simulink model "FCS_MPC_6ph_Regelungsmodell"  (R2022a)
settings: Solver=ode23t  StartTime=0.0  StopTime=0.1  RelTol=1e-3  AbsTol=1e-3  EnableMultiTasking=on
values from neighbouring files (symbols this model uses):
  f_c = 100000    [MPC_params.m]
  L_d = 2e-3    (= 0.002)    [MPC_params.m]
  L_q = 6.4e-3    (= 0.0064)    [MPC_params.m]
  L_x = 3e-3    (= 0.003)    [MPC_params.m]
  L_y = L_x    (= 0.003)    [MPC_params.m]
  p = 5    [MPC_params.m]
  psi_pm = 0.19    [MPC_params.m]
  R_ph = 0.19    [MPC_params.m]
  T_100MHz = 1/f_100MHz    (= 1e-08)    [MPC_params.m]
  u_dc = 565    [MPC_params.m]
libraries: nesl_utility x39, fl_lib x32, ee_lib x12, simulink x4, hdlsllib x3, spsAlphaBetaZerotodq0Lib x1
(part 2 of 2)

== matlab function FCS_MPC_6ph_Regelungsmodell/Microcontroller Software/Subsystem5/MATLAB Function1 ==
  data: I input; next_switching_state output
function next_switching_state = fcn(I)

    % Possible switching states of the 6-Phase 2-level inverter
    possible_swichting_states = [0	1	0	1	0	1	0	1	0	1	0	1;
                                1	0	0	1	0	1	0	1	0	1	0	1;
                                0	1	1	0	0	1	0	1	0	1	0	1;
                                1	0	1	0	0	1	0	1	0	1	0	1;
                                0	1	0	1	1	0	0	1	0	1	0	1;
                                1	0	0	1	1	0	0	1	0	1	0	1;
                                0	1	1	0	1	0	0	1	0	1	0	1;
                                1	0	1	0	1	0	0	1	0	1	0	1;
                                0	1	0	1	0	1	1	0	0	1	0	1;
                                1	0	0	1	0	1	1	0	0	1	0	1;
                                0	1	1	0	0	1	1	0	0	1	0	1;
                                1	0	1	0	0	1	1	0	0	1	0	1;
                                0	1	0	1	1	0	1	0	0	1	0	1;
                                1	0	0	1	1	0	1	0	0	1	0	1;
                                0	1	1	0	1	0	1	0	0	1	0	1;
                                1	0	1	0	1	0	1	0	0	1	0	1;
                                0	1	0	1	0	1	0	1	1	0	0	1;
                                1	0	0	1	0	1	0	1	1	0	0	1;
                                0	1	1	0	0	1	0	1	1	0	0	1;
                                1	0	1	0	0	1	0	1	1	0	0	1;
                                0	1	0	1	1	0	0	1	1	0	0	1;
                                1	0	0	1	1	0	0	1	1	0	0	1;
                                0	1	1	0	1	0	0	1	1	0	0	1;
                                1	0	1	0	1	0	0	1	1	0	0	1;
                                0	1	0	1	0	1	1	0	1	0	0	1;
                                1	0	0	1	0	1	1	0	1	0	0	1;
                                0	1	1	0	0	1	1	0	1	0	0	1;
                                1	0	1	0	0	1	1	0	1	0	0	1;
                                0	1	0	1	1	0	1	0	1	0	0	1;
                                1	0	0	1	1	0	1	0	1	0	0	1;
                                0	1	1	0	1	0	1	0	1	0	0	1;
                                1	0	1	0	1	0	1	0	1	0	0	1;
                                0	1	0	1	0	1	0	1	0	1	1	0;
                                1	0	0	1	0	1	0	1	0	1	1	0;
                                0	1	1	0	0	1	0	1	0	1	1	0;
                                1	0	1	0	0	1	0	1	0	1	1	0;
                                0	1	0	1	1	0	0	1	0	1	1	0;
                                1	0	0	1	1	0	0	1	0	1	1	0;
                                0	1	1	0	1	0	0	1	0	1	1	0;
                                1	0	1	0	1	0	0	1	0	1	1	0;
                                0	1	0	1	0	1	1	0	0	1	1	0;
                                1	0	0	1	0	1	1	0	0	1	1	0;
                                0	1	1	0	0	1	1	0	0	1	1	0;
                                1	0	1	0	0	1	1	0	0	1	1	0;
                                0	1	0	1	1	0	1	0	0	1	1	0;
                                1	0	0	1	1	0	1	0	0	1	1	0;
                                0	1	1	0	1	0	1	0	0	1	1	0;
                                1	0	1	0	1	0	1	0	0	1	1	0;
                                0	1	0	1	0	1	0	1	1	0	1	0;
                                1	0	0	1	0	1	0	1	1	0	1	0;
                                0	1	1	0	0	1	0	1	1	0	1	0;
                                1	0	1	0	0	1	0	1	1	0	1	0;
                                0	1	0	1	1	0	0	1	1	0	1	0;
                                1	0	0	1	1	0	0	1	1	0	1	0;
                                0	1	1	0	1	0	0	1	1	0	1	0;
                                1	0	1	0	1	0	0	1	1	0	1	0;
                                0	1	0	1	0	1	1	0	1	0	1	0;
                                1	0	0	1	0	1	1	0	1	0	1	0;
                                0	1	1	0	0	1	1	0	1	0	1	0;
                                1	0	1	0	0	1	1	0	1	0	1	0;
                                0	1	0	1	1	0	1	0	1	0	1	0;
                                1	0	0	1	1	0	1	0	1	0	1	0;
                                0	1	1	0	1	0	1	0	1	0	1	0;
                                1	0	1	0	1	0	1	0	1	0	1	0];

    % Initial condition
    if I==0
        I=int32(1);
    end

    % Output switching state
    next_switching_state=boolean(possible_swichting_states(I,:))';

end

== matlab function FCS_MPC_6ph_Regelungsmodell/6ph_PMSM_30deg_VSD1 ==
  data: u1 input; y1 output; u2 input; u3 input; u4 input; u5 input; u6 input; y2 output; y3 output; y4 output; y5 output; y6 output; k6 input; c6 input
function [y1,y2,y3,y4,y5,y6] = VSD_asymm_30(u1,u2,u3,u4,u5,u6,k6,c6)

A =single([0 0 0 0 0 0]');

A =    k6*[1    -0.5        -0.5        sqrt(3)/2   -sqrt(3)/2  0 ;
           0    sqrt(3)/2   -sqrt(3)/2  0.5         0.5         -1;
           1    -0.5        -0.5        -sqrt(3)/2  sqrt(3)/2   0 ;
           0    -sqrt(3)/2  sqrt(3)/2   0.5         0.5         -1;
           c6   c6          c6          0           0           0 ;
           0    0           0           c6          c6          c6] * [u1 u2 u3 u4 u5 u6]';

y1 =single(A(1));
y2 =single(A(2));
y3 =single(A(3));
y4 =single(A(4));
y5 =single(A(5));
y6 =single(A(6));

== matlab function FCS_MPC_6ph_Regelungsmodell/Microcontroller Software/Subsystem3/MATLAB Function ==
  data: i_x input; i_y input; i_d input; i_q input; Rs input; Ld input; Lq input; theta_el input; psiPM input; omega_el input; id_ref input; iq_ref input; ix_ref input; iy_ref input; u_dc_link input; SampleTime_div_Ld input; SampleTime_div_Lq input; SampleTime_div_Lx input; SampleTime_div_Ly input; J output size=[64,1]; vk input; v output size=[4,64]; id_k_1 output size=1; iq_k_1 output; ix_k_1 output size=1; iy_k_1 output
function [J,v,id_k_1,iq_k_1,ix_k_1,iy_k_1]=FCS_MPC_6Phase_PMSM_with_delay_compensation(i_x, i_y, i_d, i_q, Rs, Ld, Lq, theta_el, psiPM, omega_el, id_ref, iq_ref, ix_ref, iy_ref, u_dc_link, SampleTime_div_Ld, SampleTime_div_Lq, SampleTime_div_Lx, SampleTime_div_Ly, vk )

    % Applying Dimension of the Cost-Function Vector
    J = single(zeros(64,1));

    % Swichtingstates factors alpha beta x y
    Factors_alpha_beta_x_y = single([0	    0.333333333333333	-0.166666666666667	 0.166666666666667	-0.166666666666667	 0.166666666666667	-0.333333333333333	0	 0.288675134594813	0.622008467928146	 0.122008467928146  	0.455341801261480	 0.122008467928146	 0.455341801261480	-0.0446581987385205  0.288675134594813	-0.288675134594813	0.0446581987385205	-0.455341801261480	-0.122008467928146	-0.455341801261480	-0.122008467928146	-0.622008467928146	-0.288675134594813	0	                0.333333333333333	-0.166666666666667  	0.166666666666667	-0.166666666666667	 0.166666666666667	 -0.333333333333333	0	                 0	                 0.333333333333333	-0.166666666666667	  0.166666666666667	    -0.166666666666667	  0.166666666666667	    -0.333333333333333	 0	                 0.288675134594813	 0.622008467928146	 0.122008467928146	 0.455341801261480	 0.122008467928146	 0.455341801261480	-0.0446581987385205  0.288675134594813	-0.288675134594813	 0.0446581987385205  -0.455341801261480	  -0.122008467928146	-0.455341801261480	-0.122008467928146	-0.622008467928146	-0.288675134594813	0	0.333333333333333	-0.166666666666667	 0.166666666666667	-0.166666666666667	 0.166666666666667	-0.333333333333333	0;
                                     0	    0                    0.288675134594813	 0.288675134594813	-0.288675134594813	-0.288675134594813	 0	                0	 0.166666666666667	0.166666666666667	 0.455341801261480  	0.455341801261480	-0.122008467928146	-0.122008467928146	 0.166666666666667	 0.166666666666667	 0.166666666666667	0.166666666666667	 0.455341801261480   0.455341801261480	-0.122008467928146	-0.122008467928146	 0.166666666666667	 0.166666666666667	0.333333333333333	0.333333333333333	 0.622008467928146	    0.622008467928146	 0.0446581987385205	 0.0446581987385205	  0.333333333333333	0.333333333333333	-0.333333333333333	-0.333333333333333	-0.0446581987385205	 -0.0446581987385205	-0.622008467928146	 -0.622008467928146	    -0.333333333333333	-0.333333333333333	-0.166666666666667	-0.166666666666667	 0.122008467928146	 0.122008467928146	-0.455341801261480	-0.455341801261480	-0.166666666666667	-0.166666666666667	-0.166666666666667	-0.166666666666667	  0.122008467928146	   0.122008467928146	-0.455341801261480	-0.455341801261480	-0.166666666666667	-0.166666666666667	0	0	                 0.288675134594813	 0.288675134594813	-0.288675134594813	-0.288675134594813	 0	                0;
                                     0	    0.333333333333333	-0.166666666666667	 0.166666666666667	-0.166666666666667	 0.166666666666667	-0.333333333333333	0	-0.288675134594813	0.0446581987385205	-0.455341801261480	   -0.122008467928146	-0.455341801261480	-0.122008467928146	-0.622008467928146	-0.288675134594813	 0.288675134594813	0.622008467928146	 0.122008467928146	 0.455341801261480   0.122008467928146	 0.455341801261480	-0.0446581987385205	 0.288675134594813	0	                0.333333333333333	-0.166666666666667	    0.166666666666667	-0.166666666666667	 0.166666666666667	 -0.333333333333333	0	                 0	                 0.333333333333333	-0.166666666666667	  0.166666666666667	    -0.166666666666667	  0.166666666666667	    -0.333333333333333	 0	                -0.288675134594813	 0.0446581987385205	-0.455341801261480	-0.122008467928146	-0.455341801261480	-0.122008467928146	-0.622008467928146	-0.288675134594813	 0.288675134594813	 0.622008467928146	  0.122008467928146	   0.455341801261480	 0.122008467928146	 0.455341801261480	-0.0446581987385205  0.288675134594813	0	0.333333333333333	-0.166666666666667	 0.166666666666667	-0.166666666666667	 0.166666666666667	-0.333333333333333	0;
                                     0	    0	                -0.288675134594813	-0.288675134594813	 0.288675134594813	 0.288675134594813	 0              	0	 0.166666666666667	0.166666666666667	-0.122008467928146     -0.122008467928146	 0.455341801261480	 0.455341801261480	 0.166666666666667	 0.166666666666667	 0.166666666666667	0.166666666666667	-0.122008467928146	-0.122008467928146	 0.455341801261480	 0.455341801261480	 0.166666666666667	 0.166666666666667	0.333333333333333	0.333333333333333	 0.0446581987385205 	0.0446581987385205	 0.622008467928146	 0.622008467928146	  0.333333333333333	0.333333333333333	-0.333333333333333	-0.333333333333333	-0.622008467928146	 -0.622008467928146	    -0.0446581987385205	 -0.0446581987385205	-0.333333333333333	-0.333333333333333	-0.166666666666667	-0.166666666666667	-0.455341801261480	-0.455341801261480	 0.122008467928146	 0.122008467928146	-0.166666666666667	-0.166666666666667	-0.166666666666667	-0.166666666666667	 -0.455341801261480	  -0.455341801261480	 0.122008467928146	 0.122008467928146	-0.166666666666667	-0.166666666666667	0	0	                -0.288675134594813	-0.288675134594813	 0.288675134594813	 0.288675134594813	 0	                0]);
    
    % Park-Transformation of the switchingstates factors
    B = single([0 0]');
    Factors_d_q_x_y =single(zeros (4,64));
    Factors_d_q_x_y(3,:) = Factors_alpha_beta_x_y(3,:);
    Factors_d_q_x_y(4,:) = Factors_alpha_beta_x_y(4,:);
    cos_theta_el = single(cos(theta_el));
    sin_theta_el = single(sin(theta_el));
    for i=1:64
        B =single([cos_theta_el         sin_theta_el;
                   -sin_theta_el        cos_theta_el] * [Factors_alpha_beta_x_y(1,i) Factors_alpha_beta_x_y(2,i)]');
        Factors_d_q_x_y(1,i) = B(1);
        Factors_d_q_x_y(2,i) = B(2);
    end
    
    %Calculation of the voltages per switching state in alpha beta coordinates
    v = single(u_dc_link*Factors_d_q_x_y);

    % Delay compensation with a modell of a 6-Phase-PMSM
    id_k_1 = single(SampleTime_div_Ld*(vk(1)-i_d*Rs+omega_el*Lq*i_q)+i_d);
    iq_k_1 = single(SampleTime_div_Lq*(vk(2)-i_q*Rs-omega_el*(psiPM+i_d*Ld))+i_q);
    ix_k_1 = single(SampleTime_div_Lx*(vk(3)-i_x*Rs)+i_x);
    iy_k_1 = single(SampleTime_div_Ly*(vk(4)-i_y*Rs)+i_y);

    for i=1:64
        % Prediction of the d-, q-, x-, y-currents of the 6-Phase-PMSM with the finite control set 
        id_k_2 = single(SampleTime_div_Ld*(v(1,i)-id_k_1*Rs+omega_el*Lq*iq_k_1)+id_k_1);
        iq_k_2 = single(SampleTime_div_Lq*(v(2,i)-iq_k_1*Rs-omega_el*(psiPM+id_k_1*Ld))+iq_k_1);
        ix_k_2 = single(SampleTime_div_Lx*(v(3,i)-ix_k_1*Rs)+ix_k_1);
        iy_k_2 = single(SampleTime_div_Ly*(v(4,i)-iy_k_1*Rs)+iy_k_1);
        
        % Calculation of the cost function
        J(i) = single((id_ref-id_k_2)^2+(iq_ref-iq_k_2)^2+(ix_ref-ix_k_2)^2+(iy_ref-iy_k_2)^2);
    end
   
end

== matlab function FCS_MPC_6ph_Regelungsmodell/Microcontroller Software/Subsystem2/6ph_PMSM_30deg_VSD1 ==
  data: i_a1 input; i_alpha output; i_b1 input; i_c1 input; i_a2 input; i_b2 input; i_c2 input; theta_el input; i_beta output; i_x output; i_y output; i_0_plus output; i_0_minus output; i_d output; i_q output
function [i_alpha,i_beta,i_x,i_y,i_0_plus,i_0_minus,i_d,i_q] = VSD_and_Park_transformation(i_a1,i_b1,i_c1,i_a2,i_b2,i_c2,theta_el)

    % VSD-Transformation
    A =[0 0 0 0 0 0]';

    A =    (1/3)*[1    -0.5        -0.5        sqrt(3)/2   -sqrt(3)/2  0 ;
                  0    sqrt(3)/2   -sqrt(3)/2  0.5         0.5         -1;
                  1    -0.5        -0.5        -sqrt(3)/2  sqrt(3)/2   0 ;
                  0    -sqrt(3)/2  sqrt(3)/2   0.5         0.5         -1;
                  1    1           1           0           0           0 ;
                  0    0           0           1           1           1] * [i_a1 i_b1 i_c1 i_a2 i_b2 i_c2]';

    i_alpha = A(1);
    i_beta = A(2);
    i_x = A(3);
    i_y = A(4);
    i_0_plus = A(5);
    i_0_minus = A(6);

    % Park-Transformation

    B = [0 0]';

     B = [cos(theta_el)       sin(theta_el);
         -sin(theta_el)       cos(theta_el)] * [i_alpha i_beta]';

    i_d = B(1);
    i_q = B(2);

end

== matlab function FCS_MPC_6ph_Regelungsmodell/Microcontroller Software/Subsystem3/MATLAB Function1 ==
  data: J input; I output; v input; v_opt output
function [I,v_opt] = Optimal_Value(J,v)

    % Determination of the index of the minimum of the cost function vector
    min = J(1);
    I = int32(1);
    for i = int32(2):int32(64)
        if J(i)<min
            I = i;
            min = J(i);
        end
    end

    % Output of the determined voltages (d, q, x, y) v_opt respectively vk
    v_opt = single(zeros(4,1));
    for i=1:4
        v_opt(i) = v(i,I);
    end

end
